simulink model "Kc_donghocthuan"  (R2022b)
settings: Solver=FixedStepAuto  StartTime=0.0  StopTime=10.0  FixedStep=0.01  RelTol=1e-3
settings Model: Creator=Admin  LastModifiedBy=Admin

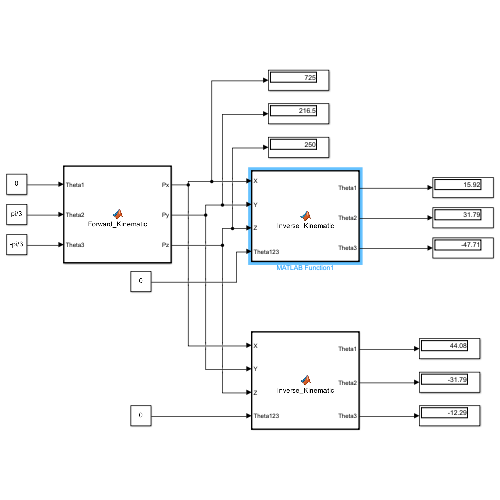
[thumbnail: Simulink's stored preview of the top-level diagram]
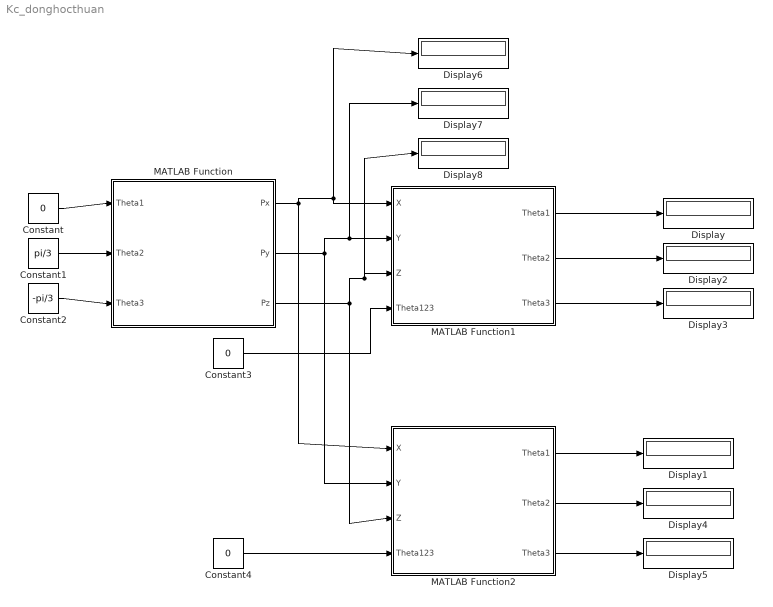
== system Kc_donghocthuan ==
  Constant : Constant  Value=0
  Constant1 : Constant  Value=pi/3
  Constant2 : Constant  Value=-pi/3
  Constant3 : Constant  Value=0
  Constant4 : Constant  Value=0
  Display{,1..8} (9 alike) : Display
  MATLAB Function : MATLAB Function  TreatAsAtomicUnit=on
  MATLAB Function1 : MATLAB Function  TreatAsAtomicUnit=on
  MATLAB Function2 : MATLAB Function  TreatAsAtomicUnit=on
  wires:
  Constant2/1 -> MATLAB Function/3(Theta3)
  Constant1/1 -> MATLAB Function/2(Theta2)
  Constant/1 -> MATLAB Function/1(Theta1)
  Constant3/1 -> MATLAB Function1/4(Theta123)
  Constant4/1 -> MATLAB Function2/4(Theta123)
  MATLAB Function1/1(Theta1) -> Display/1
  MATLAB Function1/2(Theta2) -> Display2/1
  MATLAB Function1/3(Theta3) -> Display3/1
  MATLAB Function2/1(Theta1) -> Display1/1
  MATLAB Function2/2(Theta2) -> Display4/1
  MATLAB Function2/3(Theta3) -> Display5/1
  MATLAB Function/3(Pz) -> MATLAB Function2/3(Z), Display8/1, MATLAB Function1/3(Z)
  MATLAB Function/2(Py) -> MATLAB Function2/2(Y), Display7/1, MATLAB Function1/2(Y)
  MATLAB Function/1(Px) -> MATLAB Function2/1(X), Display6/1, MATLAB Function1/1(X)

== matlab function Kc_donghocthuan/MATLAB Function1 ==
  data: X input; Theta1 output; Y input; Theta2 output; Theta3 output; Z input; Theta123 input
function [Theta1,Theta2,Theta3] = Inverse_Kinematic(X,Y,Z,Theta123)
L1 = 200; L2 = 250; L3 = 200; L4 = 150;
%% Tinh theta 2
N = X - L1 - L4*cosd(Theta123);
M = Y - L4*sind(Theta123);
C_T2 = (N^2 + M^2 - L2^2 - L3^2) / (2*L2*L3);
S_T2 = sqrt(abs(1 - C_T2^2));
Theta2 = atan2d(S_T2,C_T2);

%% Tinh theta 1
C_T1 = (N*(L2+L3*cosd(Theta2)) + M*L3*sind(Theta2)) / (L2^2+2*L2*L3*cosd(Theta2)+L3^2);
S_T1 = (M*(L2+L3*cosd(Theta2)) - N*L3*sind(Theta2)) / (L2^2+2*L2*L3*cosd(Theta2)+L3^2);
Theta1 = atan2d(S_T1,C_T1);

%% Tinh theta 3
Theta3 = Theta123 - Theta1 - Theta2;

== matlab function Kc_donghocthuan/MATLAB Function ==
  data: Theta1 input; Px output; Theta2 input; Theta3 input; Py output; Pz output
function [Px,Py,Pz] = Forward_Kinematic(Theta1,Theta2,Theta3)
%% TINH DONG HOC THUAN CHO ROBOT
% khai bao thong so cho Robot
L0 = 100; L1 = 200; L2 = 250; L3 = 250; L4 = 150; d = 30;
%Ma tran chuyen doi tu he 0 sang 1
T01 = [cos(Theta1), -sin(Theta1), 0, L1;
       sin(Theta1),  cos(Theta1), 0,  0;
                  0,             0, 1, L0+3*d;
                  0,             0, 0,  1];
%Ma tran chuyen doi tu he 1 sang 2
T12 = [cos(Theta2), -sin(Theta2), 0, L2;
       sin(Theta2),  cos(Theta2), 0,  0;
                  0,             0, 1,  d;
                  0,             0, 0,  1];
%Ma tran chuyen doi tu he 2 sang 3
T23 = [cos(Theta3), -sin(Theta3), 0, L3
       sin(Theta3),  cos(Theta3), 0,  0
                  0,             0, 1,  d
                  0,             0, 0,  1];
%Ma tran chuyen doi tu he 2 sang 3
T34 = [1, 0, 0, L4
       0, 1, 0,  0
       0, 0, 1,  0
       0, 0, 0,  1];
% Ma tran chuyen doi sau cung
T04 = T01 * T12 * T23 * T34;
% Tính vị trí cho ROBOT
Px=T04(1,4);
Py=T04(2,4);
Pz=T04(3,4);

== matlab function Kc_donghocthuan/MATLAB Function2 ==
  data: X input; Theta1 output; Y input; Theta2 output; Theta3 output; Z input; Theta123 input
function [Theta1,Theta2,Theta3] = Inverse_Kinematic(X,Y,Z,Theta123)
L1 = 200; L2 = 250; L3 = 200; L4 = 150;
%% Tinh theta 2
N = X - L1 - L4*cosd(Theta123);
M = Y - L4*sind(Theta123);
C_T2 = (N^2 + M^2 - L2^2 - L3^2) / (2*L2*L3);
S_T2 = -sqrt(abs(1 - C_T2^2));
Theta2 = atan2d(S_T2,C_T2);

%% Tinh theta 1
C_T1 = (N*(L2+L3*cosd(Theta2)) + M*L3*sind(Theta2)) / (L2^2+2*L2*L3*cosd(Theta2)+L3^2);
S_T1 = (M*(L2+L3*cosd(Theta2)) - N*L3*sind(Theta2)) / (L2^2+2*L2*L3*cosd(Theta2)+L3^2);
Theta1 = atan2d(S_T1,C_T1);

%% Tinh theta 3
Theta3 = Theta123 - Theta1 - Theta2;
